simulink model "mpcController"  (R2022a)
settings: Solver=ode5  StartTime=0.0  StopTime=inf  RelTol=1e-3
values from neighbouring files (symbols this model uses):
  A_full = zeros(nX * (nH + 1), nX)    [controllerInit.m]
  B_full = zeros(nX * nH, nU * nH)    [controllerInit.m]
  lb_u_full = ub_u_full    [controllerInit.m]
  lb_x_full = ub_x_full    [controllerInit.m]
  opts = readyFamiliarisation(opts)    [main.m]
  R_full = zeros(nU * nH)    [controllerInit.m]
  ub_u_full = zeros(nU * nH, 1)    [controllerInit.m]
  ub_x_full = zeros(nX * (nH + 1), 1)    [controllerInit.m]
undefined symbols (not defined in the file or in its folder): C_full, QstructInitial, R_full_zeros, Serial_Port, simulinkStructInitial, Standard_Devices, UDP_Protocol
libraries: sldrtlib x5, simulink_extras x1, sharedtransform x1
settings Model: PacingRate=0.350000  Creator=simonas  LastModifiedBy=Simonas
settings HardwareCC: ProdBitPerLong=64  ProdHWDeviceType=Intel->x86-64 (Linux 64)
settings RTWCC: Description=Simulink Desktop Real-Time  SystemTargetFile=sldrt.tlc  TemplateMakefile=sldrt.tmf  RTWCompilerOptimization=on
settings CodeAppCC: MaxIdLength=95
settings SimulinkDesktopRealTimeCC: TargetLibSuffix=_sldrt.a  TargetPreCompLibLocation=C:\Program Files\MATLAB\R2022a\toolbox\sldrt\lib\win64

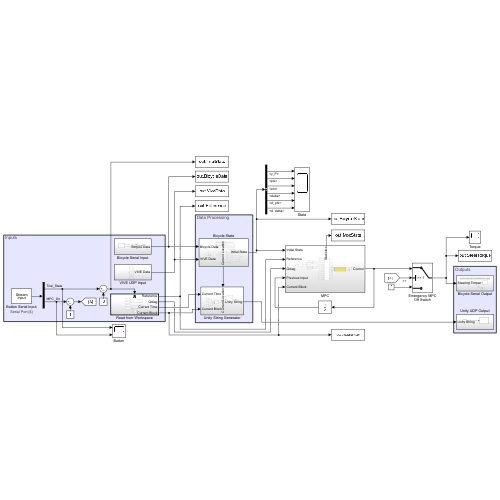
[thumbnail: Simulink's stored preview of the top-level diagram]
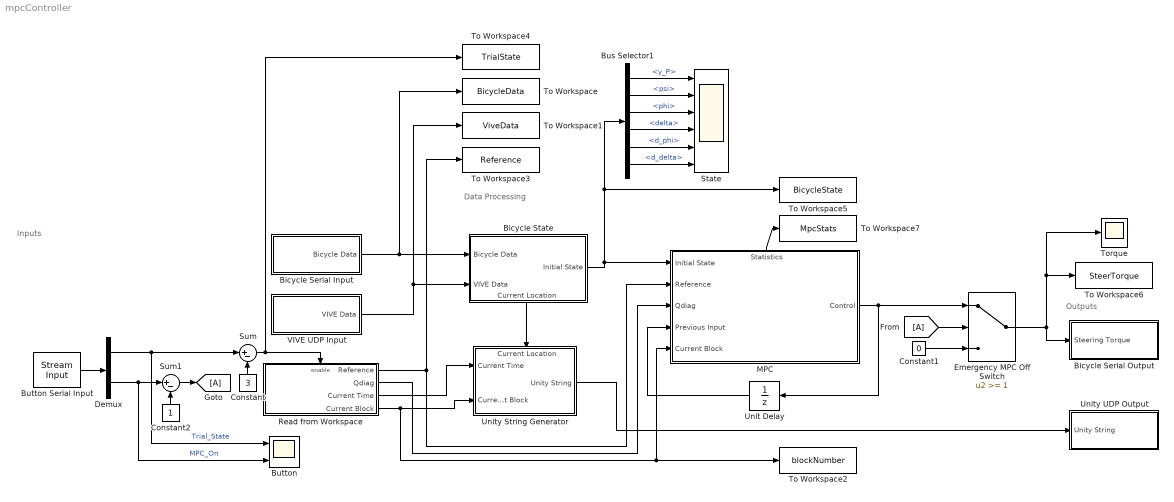
== system mpcController ==
  note: Inputs
  note: Data Processing
  note: Outputs
  Bicycle Serial Input : Subsystem
  Bicycle Serial Output : Subsystem
  Bicycle State : Subsystem
      settings: PortSchema="{\"entries\":[{\"content\":{\"sides\":[{\"content\":{\"connectorIds\":[\"In1\",\"In2\"]},\"type\":\"ConnectorPlacement.EquallySpacedRectSide\",\"uuid\":\"c5d89f74-e35e-400b-a49a-6a7c3bbb3cee\"},{\"content\":{\"connectorIds\":[\"Out1\"],\"side\":\"RIGHT\"},\"type\":\"ConnectorPlacement.EquallySpacedRectSide\",\"uuid\":\"d3946c1d-493c-4283-9feb-9c130facb0a9\"},{\"content\":{\"connectorIds\":[],\"side\":\"TOP\"},\"type\":\"ConnectorPlacement.EquallySpacedRectSide\",\"uuid\":\"f7eeef6e-15d0-4138-b893-66df70237323\"},{\"content\":{\"connectorIds\":[\"Out2\"],\"side\":\"BOTTOM\"},\"type\":\"ConnectorPlacement.EquallySpacedRectSide\",\"uuid\":\"d8cc5cfa-3fb7-476d-9b2c-860b356f327e\"}]},\"type\":\"ConnectorPlacement.EquallySpacedConnector\",\"uuid\":\"85360968-76db-44cc-98f9-7355ff2a9269\"}],\"packageUris\":[\"http://schema.mathworks.com/mf0/Connector/R2020b\"],\"version\":\"1.0\"}"
  Bus Selector1 : BusSelector  OutputSignals=y_P,psi,phi,delta,d_phi,d_delta
  Button : Scope  NumInputPorts=2
  Button Serial Input : sldrtlib/Stream Input  SampleTime=0.025  MaxMissedTicks=1000000  ShowMissedTicks=off  YieldWhenWaiting=off  DrvName=Standard_Devices/Serial_Port  DrvAddress=4  DrvOptions=[115200 8 0 0 0 0 0 0]  DataTypes='2*int32'  FormatString='%d,%d'  Terminator={'\n', '\r'}  ShowReady=off  ShowError=off
      settings: AttributesFormatString=Serial Port [4]  SourceProductBaseCode=WT
  Constant : Constant  Value=3
  Constant1 : Constant  Value=0  SampleTime=opts.Ts_mpc
  Constant2 : Constant
  Demux : Demux  Outputs=2
  Emergency MPC Off Switch : Switch  Threshold=1  SaturateOnIntegerOverflow=off  InputSameDT=off
  From : From
  Goto : Goto
  MPC : Subsystem
      settings: PortSchema="{\"entries\":[{\"content\":{\"sides\":[{\"content\":{\"connectorIds\":[\"In1\",\"In2\",\"In3\",\"In4\",\"In5\"]},\"type\":\"ConnectorPlacement.EquallySpacedRectSide\",\"uuid\":\"837940b0-492f-49e7-ad78-2f53a96cfdb0\"},{\"content\":{\"connectorIds\":[\"Out1\"],\"side\":\"RIGHT\"},\"type\":\"ConnectorPlacement.EquallySpacedRectSide\",\"uuid\":\"0b454771-57c7-4798-97e4-6e41a25b36dc\"},{\"content\":{\"connectorIds\":[\"Out2\"],\"side\":\"TOP\"},\"type\":\"ConnectorPlacement.EquallySpacedRectSide\",\"uuid\":\"d0d77e63-f0c6-441e-9a4a-b6dfb0057ad2\"},{\"content\":{\"connectorIds\":[],\"side\":\"BOTTOM\"},\"type\":\"ConnectorPlacement.EquallySpacedRectSide\",\"uuid\":\"b6921f02-8dc3-4ff1-8cb0-61ac83bc5ab1\"}]},\"type\":\"ConnectorPlacement.EquallySpacedConnector\",\"uuid\":\"6905a0a5-9fd3-4ab9-9143-61679843e617\"}],\"packageUris\":[\"http://schema.mathworks.com/mf0/Connector/R2020b\"],\"version\":\"1.0\"}"
  Read from Workspace : Subsystem  TreatAsAtomicUnit=on
  State : Scope  NumInputPorts=6
  Sum : Sum  Inputs=|+-
  Sum1 : Sum  Inputs=|+-
  To Workspace : ToWorkspace  VariableName=BicycleData  SaveFormat=Timeseries  SampleTime=-1
  To Workspace1 : ToWorkspace  VariableName=ViveData  SaveFormat=Timeseries  SampleTime=-1
  To Workspace2 : ToWorkspace  VariableName=blockNumber  SaveFormat=Timeseries  SampleTime=-1
  To Workspace3 : ToWorkspace  VariableName=Reference  SaveFormat=Timeseries  SampleTime=-1
  To Workspace4 : ToWorkspace  VariableName=TrialState  SaveFormat=Timeseries  SampleTime=-1
  To Workspace5 : ToWorkspace  VariableName=BicycleState  SaveFormat=Timeseries  SampleTime=-1
  To Workspace6 : ToWorkspace  VariableName=SteerTorque  SaveFormat=Timeseries  SampleTime=-1
  To Workspace7 : ToWorkspace  VariableName=MpcStats  SaveFormat=Timeseries  SampleTime=-1
  Torque : Scope
  Unit Delay : UnitDelay  SampleTime=opts.Ts_mpc  HasFrameUpgradeWarning=on
  Unity String Generator : Subsystem
      settings: PortSchema="{\"entries\":[{\"content\":{\"sides\":[{\"content\":{\"connectorIds\":[\"In1\",\"In2\"]},\"type\":\"ConnectorPlacement.EquallySpacedRectSide\",\"uuid\":\"995dcb62-78f8-423c-99d5-aa9c538d86ef\"},{\"content\":{\"connectorIds\":[\"Out1\"],\"side\":\"RIGHT\"},\"type\":\"ConnectorPlacement.EquallySpacedRectSide\",\"uuid\":\"d6e446ff-77b4-4bca-8c68-e505a29969fe\"},{\"content\":{\"connectorIds\":[\"In3\"],\"side\":\"TOP\"},\"type\":\"ConnectorPlacement.EquallySpacedRectSide\",\"uuid\":\"a2ee3f9a-5385-4b4c-abf0-7e00a59d14cf\"}]},\"type\":\"ConnectorPlacement.EquallySpacedConnector\",\"uuid\":\"6b026230-ac01-4f6d-82d7-753dc9fb2975\"}],\"packageUris\":[\"http://schema.mathworks.com/mf0/Connector/R2020b\"],\"version\":\"1.0\"}"
  Unity UDP Output : Subsystem
  VIVE UDP Input : Subsystem
  wires:
  Bicycle Serial Input/1(Bicycle Data) -> Bicycle State/1(Bicycle Data), To Workspace/1
  VIVE UDP Input/1(VIVE Data) -> Bicycle State/2(VIVE Data), To Workspace1/1
  Bicycle State/2(Current Location) -> Unity String Generator/3(Current Location)
  Bicycle State/1(Initial State) -> Bus Selector1/1, To Workspace5/1, MPC/1(Initial State)
  Demux/1 -> Sum/1, Button/1  "Trial_State"
  Button Serial Input/1 -> Demux/1
  Sum/1 -> To Workspace4/1, Read from Workspace/Enable
  Constant/1 -> Sum/2
  From/1 -> Emergency MPC Off Switch/2
  Constant1/1 -> Emergency MPC Off Switch/3
  Emergency MPC Off Switch/1 -> Bicycle Serial Output/1(Steering Torque), Torque/1, To Workspace6/1
  Sum1/1 -> Goto/1
  Constant2/1 -> Sum1/2
  Demux/2 -> Button/2, Sum1/1  "MPC_On"
  Read from Workspace/3(Current Time) -> Unity String Generator/1(Current Time)
  Read from Workspace/1(Reference) -> To Workspace3/1, MPC/2(Reference)
  Read from Workspace/2(Qdiag) -> MPC/3(Qdiag)
  MPC/2(Statistics) -> To Workspace7/1
  Unit Delay/1 -> MPC/4(Previous Input)
  Unity String Generator/1(Unity String) -> Unity UDP Output/1(Unity String)
  Bus Selector1/1 -> State/1  "<y_P>"
  Bus Selector1/3 -> State/3  "<phi>"
  Bus Selector1/4 -> State/4  "<delta>"
  Bus Selector1/2 -> State/2  "<psi>"
  Bus Selector1/5 -> State/5  "<d_phi>"
  Bus Selector1/6 -> State/6  "<d_delta>"
  MPC/1(Control) -> Emergency MPC Off Switch/1, Unit Delay/1
  Read from Workspace/4(Current Block) -> Unity String Generator/2(Current Block), MPC/5(Current Block), To Workspace2/1

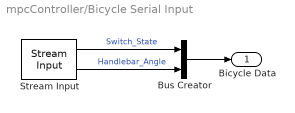
== system mpcController/Bicycle Serial Input ==
  Bus Creator : BusCreator  Inputs=2
  Stream Input : sldrtlib/Stream Input  SampleTime=opts.Ts_ser  MaxMissedTicks=1000000  ShowMissedTicks=off  YieldWhenWaiting=on  DrvName=Standard_Devices/Serial_Port  DrvAddress=3  DrvOptions=[115200 8 0 0 0 0 0 0]  DataTypes={'uint8','double'}  FormatString='%d,%f'  Terminator={'\n'}  ShowReady=off  ShowError=off
      settings: AttributesFormatString=Serial Port [3]  SourceProductBaseCode=WT
  Bicycle Data : Outport
  wires:
  Stream Input/1 -> Bus Creator/1  "Switch_State"
  Stream Input/2 -> Bus Creator/2  "Handlebar_Angle"
  Bus Creator/1 -> Bicycle Data/1

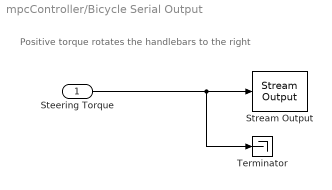
== system mpcController/Bicycle Serial Output ==
  note: Positive torque rotates the handlebars to the right
  Steering Torque : Inport
  Stream Output : sldrtlib/Stream Output  SampleTime=opts.Ts_mpc  MaxMissedTicks=1000000  ShowMissedTicks=off  YieldWhenWaiting=on  DrvName=Standard_Devices/Serial_Port  DrvAddress=3  DrvOptions=[115200 8 0 0 0 0 0 0]  PortSizes=1  FormatString='%.3f\n'  ShowReady=off  ShowError=off  InitialValue=[]  FinalValue=[]
      settings: AttributesFormatString=Serial Port [3]  SourceProductBaseCode=WT
  Terminator : Terminator
  wires:
  Steering Torque/1 -> Stream Output/1, Terminator/1

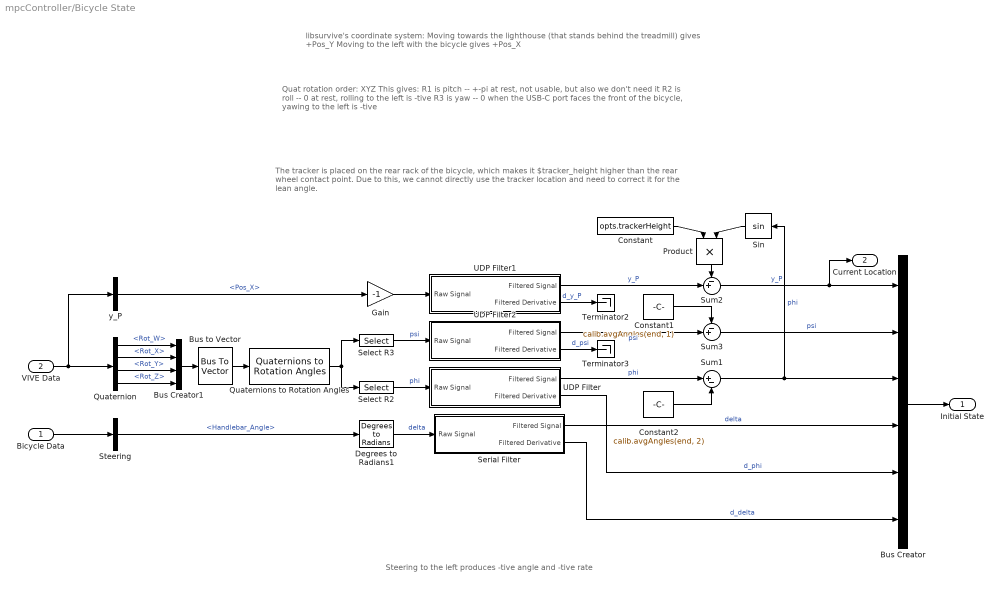
== system mpcController/Bicycle State ==
  note: The tracker is placed on the rear rack of the bicycle, which makes it $tracker_height higher than the rear wheel contact point. Due to this, we cannot directly use the tracker location and need to correct it for the lean angle.
  note: Steering to the left produces -tive angle and -tive rate
  note: libsurvive's coordinate system:
      | Moving towards the lighthouse (that stands behind the treadmill) gives +Pos_Y
      | Moving to the left with the bicycle gives +Pos_X
  note: Quat rotation order: XYZ
      | This gives:
      | R1 is pitch -- +-pi at rest, not usable, but also we don't need it
      | R2 is roll -- 0 at rest, rolling to the left is -tive
      | R3 is yaw -- 0 when the USB-C port faces the front of the bicycle, yawing to the left is -tive
  Bicycle Data : Inport
  VIVE Data : Inport  Port=2
  Bus Creator : BusCreator  Inputs=6
  Bus Creator1 : BusCreator  Inputs=4
  Bus to Vector : BusToVector
  Constant : Constant  Value=opts.trackerHeight
  Constant1 : Constant  Value=calib.avgAngles(end, 1)  SampleTime=opts.Ts_udp
  Constant2 : Constant  Value=calib.avgAngles(end, 2)  SampleTime=opts.Ts_udp
  Degrees to Radians1 : simulink_extras/Transformations/Degrees to Radians
  Gain : Gain  Gain=-1
  Product : Product
  Quaternion : BusSelector  OutputSignals=Rot_W,Rot_X,Rot_Y,Rot_Z
  Quaternions to Rotation Angles : sharedtransform/Quaternions to Rotation Angles  rotationOrder=XYZ  aMode=aMode
      settings: SourceProductBaseCode=AE,PW,DR,MT,VE
  Select R2 : Selector  InputPortWidth=3  IndexOptions=Index vector (dialog)  Indices=2  OutputSizes=1
  Select R3 : Selector  InputPortWidth=3  IndexOptions=Index vector (dialog)  Indices=3  OutputSizes=1
  Serial Filter : Subsystem
  Sin : Trigonometry
  Steering : BusSelector  OutputSignals=Handlebar_Angle
  Sum1 : Sum  Inputs=|+-
  Sum2 : Sum  Inputs=-+|
  Sum3 : Sum  Inputs=-+|
  Terminator2 : Terminator
  Terminator3 : Terminator
  UDP Filter : Subsystem
  UDP Filter1 : Subsystem
  UDP Filter2 : Subsystem
  y_P : BusSelector  OutputSignals=Pos_X
  Initial State : Outport
  Current Location : Outport  Port=2
  wires:
  VIVE Data/1 -> y_P/1, Quaternion/1
  Quaternion/2 -> Bus Creator1/2  "<Rot_X>"
  Quaternion/3 -> Bus Creator1/3  "<Rot_Y>"
  Quaternion/4 -> Bus Creator1/4  "<Rot_Z>"
  Select R2/1 -> UDP Filter/1(Raw Signal)  "phi"
  y_P/1 -> Gain/1  "<Pos_X>"
  Bicycle Data/1 -> Steering/1
  Steering/1 -> Degrees to Radians1/1  "<Handlebar_Angle>"
  Bus Creator/1 -> Initial State/1
  Quaternion/1 -> Bus Creator1/1  "<Rot_W>"
  Bus Creator1/1 -> Bus to Vector/1
  Bus to Vector/1 -> Quaternions to Rotation Angles/1
  Quaternions to Rotation Angles/1 -> Select R3/1, Select R2/1
  Degrees to Radians1/1 -> Serial Filter/1(Raw Signal)  "delta"
  Gain/1 -> UDP Filter1/1(Raw Signal)
  Constant/1 -> Product/1
  Sin/1 -> Product/2
  UDP Filter/2(Filtered Derivative) -> Bus Creator/5  "d_phi"
  Serial Filter/1(Filtered Signal) -> Bus Creator/4  "delta"
  Serial Filter/2(Filtered Derivative) -> Bus Creator/6  "d_delta"
  UDP Filter1/2(Filtered Derivative) -> Terminator2/1  "d_y_P"
  Select R3/1 -> UDP Filter2/1(Raw Signal)  "psi"
  UDP Filter2/1(Filtered Signal) -> Sum3/2  "psi"
  UDP Filter2/2(Filtered Derivative) -> Terminator3/1  "d_psi"
  UDP Filter1/1(Filtered Signal) -> Sum2/2  "y_P"
  Sum2/1 -> Current Location/1, Bus Creator/1  "y_P"
  Product/1 -> Sum2/1
  Sum1/1 -> Sin/1, Bus Creator/3  "phi"
  Sum3/1 -> Bus Creator/2  "psi"
  Constant1/1 -> Sum3/1
  UDP Filter/1(Filtered Signal) -> Sum1/1  "phi"
  Constant2/1 -> Sum1/2

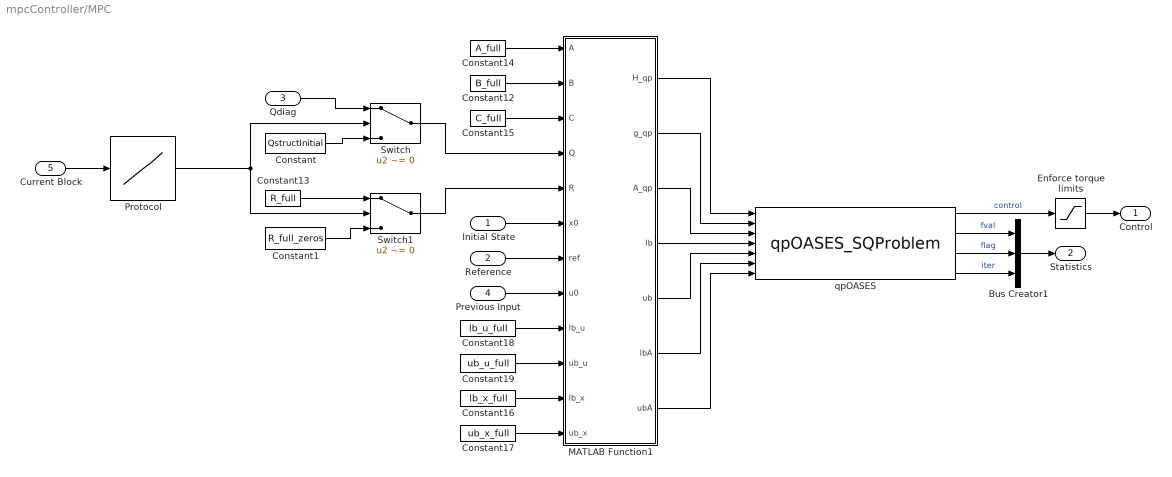
== system mpcController/MPC ==
  Initial State : Inport
  Reference : Inport  Port=2
  Qdiag : Inport  Port=3
  Previous Input : Inport  Port=4
  Current Block : Inport  Port=5
  Bus Creator1 : BusCreator  Inputs=3
  Constant : Constant  Value=QstructInitial
  Constant1 : Constant  Value=R_full_zeros  SampleTime=opts.Ts_mpc
  Constant12 : Constant  Value=B_full  SampleTime=opts.Ts_mpc
  Constant13 : Constant  Value=R_full  SampleTime=opts.Ts_mpc
  Constant14 : Constant  Value=A_full  SampleTime=opts.Ts_mpc
  Constant15 : Constant  Value=C_full  SampleTime=opts.Ts_mpc
  Constant16 : Constant  Value=lb_x_full  SampleTime=opts.Ts_mpc
  Constant17 : Constant  Value=ub_x_full  SampleTime=opts.Ts_mpc
  Constant18 : Constant  Value=lb_u_full  SampleTime=opts.Ts_mpc
  Constant19 : Constant  Value=ub_u_full  SampleTime=opts.Ts_mpc
  Enforce torque limits : Saturate  UpperLimit=opts.steerTorqueLim  LowerLimit=-opts.steerTorqueLim
  MATLAB Function1 : MATLAB Function  TreatAsAtomicUnit=on  SystemSampleTime=opts.Ts_mpc  VariantControl=Choice
  Protocol : Lookup_n-D  NumberOfTableDimensions=1  BreakpointsForDimension1=opts.lookupBreakpoints  Table=opts.lookupValues  InternalRulePriority=Speed  RndMeth=Simplest
  Switch : Switch  Criteria=u2 ~= 0  SaturateOnIntegerOverflow=off  InputSameDT=off
  Switch1 : Switch  Criteria=u2 ~= 0  SaturateOnIntegerOverflow=off  InputSameDT=off
  qpOASES : S-Function  FunctionName=qpOASES_SQProblem  SFunctionDeploymentMode=off  EnableBusSupport=off
  Control : Outport
  Statistics : Outport  Port=2
  wires:
  Enforce torque limits/1 -> Control/1
  Constant12/1 -> MATLAB Function1/2(B)
  Constant18/1 -> MATLAB Function1/9(lb_u)
  MATLAB Function1/1(H_qp) -> qpOASES/1
  Constant16/1 -> MATLAB Function1/11(lb_x)
  Constant19/1 -> MATLAB Function1/10(ub_u)
  Constant17/1 -> MATLAB Function1/12(ub_x)
  Bus Creator1/1 -> Statistics/1
  qpOASES/4 -> Bus Creator1/3  "iter"
  qpOASES/2 -> Bus Creator1/1  "fval"
  MATLAB Function1/3(A_qp) -> qpOASES/3
  Reference/1 -> MATLAB Function1/7(ref)
  qpOASES/3 -> Bus Creator1/2  "flag"
  MATLAB Function1/4(lb) -> qpOASES/4
  MATLAB Function1/2(g_qp) -> qpOASES/2
  Constant14/1 -> MATLAB Function1/1(A)
  MATLAB Function1/5(ub) -> qpOASES/5
  MATLAB Function1/7(ubA) -> qpOASES/7
  Constant15/1 -> MATLAB Function1/3(C)
  MATLAB Function1/6(lbA) -> qpOASES/6
  Previous Input/1 -> MATLAB Function1/8(u0)
  Initial State/1 -> MATLAB Function1/6(x0)
  qpOASES/1 -> Enforce torque limits/1  "control"
  Current Block/1 -> Protocol/1
  Switch/1 -> MATLAB Function1/4(Q)
  Qdiag/1 -> Switch/1
  Switch1/1 -> MATLAB Function1/5(R)
  Constant13/1 -> Switch1/1
  Protocol/1 -> Switch1/2, Switch/2
  Constant/1 -> Switch/3
  Constant1/1 -> Switch1/3

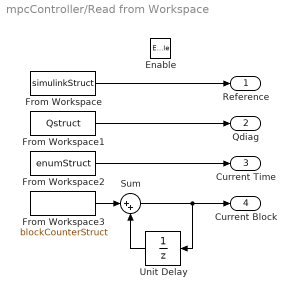
== system mpcController/Read from Workspace ==
  Enable : EnablePort  StatesWhenEnabling=reset
  From Workspace : FromWorkspace  VariableName=simulinkStruct  SampleTime=opts.Ts_mpc  Interpolate=off  OutputAfterFinalValue=Cyclic repetition
  From Workspace1 : FromWorkspace  VariableName=Qstruct  SampleTime=opts.Ts_mpc  Interpolate=off  OutputAfterFinalValue=Cyclic repetition
  From Workspace2 : FromWorkspace  VariableName=enumStruct  SampleTime=opts.Ts_mpc  Interpolate=off  OutputAfterFinalValue=Cyclic repetition
  From Workspace3 : FromWorkspace  VariableName=blockCounterStruct  SampleTime=opts.Ts_mpc  Interpolate=off  OutputAfterFinalValue=Cyclic repetition
  Sum : Sum  Inputs=|++
  Unit Delay : UnitDelay  InitialCondition=1  SampleTime=opts.Ts_mpc  HasFrameUpgradeWarning=on
  Reference : Outport  InitialOutput=simulinkStructInitial
  Qdiag : Outport  Port=2  OutputWhenDisabled=reset  InitialOutput=QstructInitial
  Current Time : Outport  Port=3  OutputWhenDisabled=reset  InitialOutput=0
  Current Block : Outport  Port=4  OutputWhenDisabled=reset  InitialOutput=1
  wires:
  From Workspace/1 -> Reference/1
  From Workspace1/1 -> Qdiag/1
  From Workspace2/1 -> Current Time/1
  From Workspace3/1 -> Sum/1
  Sum/1 -> Unit Delay/1, Current Block/1
  Unit Delay/1 -> Sum/2

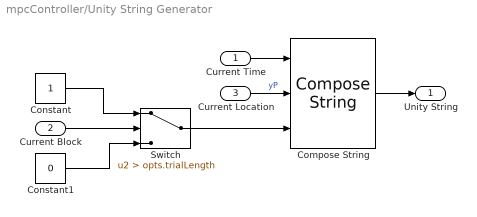
== system mpcController/Unity String Generator ==
  Current Time : Inport
  Current Block : Inport  Port=2
  Current Location : Inport  Port=3
  Compose String : ComposeString  Format="\"%.0f,%.3f,%.0f\\n\""
  Constant : Constant
  Constant1 : Constant  Value=0
  Switch : Switch  Criteria=u2 > Threshold  Threshold=opts.trialLength  SaturateOnIntegerOverflow=off  InputSameDT=off
  Unity String : Outport  OutDataTypeStr=string
  wires:
  Current Time/1 -> Compose String/1
  Current Location/1 -> Compose String/2  "yP"
  Compose String/1 -> Unity String/1
  Current Block/1 -> Switch/2
  Constant/1 -> Switch/1
  Constant1/1 -> Switch/3
  Switch/1 -> Compose String/3

== system mpcController/Unity UDP Output ==
  Unity String : Inport
  Stream Output : sldrtlib/Stream Output  SampleTime=opts.Ts_udp  MaxMissedTicks=1000000  ShowMissedTicks=off  YieldWhenWaiting=on  DrvName=Standard_Devices/UDP_Protocol  DrvAddress=8005  DrvOptions=[0 8006 49 50 55 46 48 46 48 46 49 0 0 0 0 0 0 0 0 0 0 0 0 0 0 0 0 0 0 0 0 0 0 0 0 0 0 0 0 0 0 0 0 0 0 0 0 0 0 0 0 0 0 0 0 0 0 0 0 0 0 0 0 0 0 0 0 0 0 0 0 0 0 0 0 0 0 0 0 0 0 0 0 0 0 0 0 0 0 0 0 0 0 0 0 0 0 0 0 0 0 0 0 0 0 0 0 0 0 0 0 0 0 0 0 0 0 0 0 0 0 0 0 0 0 0 0 0 0 0 0 0 0 0 0 0 0 0 0 0 0 0 0 0 0 0 0 0 0 0 0 0 0 0 0 0 0 0 0 0 0 0 0 0 0 0 0 0 0 0 0 0 0 0 0 0 0 0 0 0 0 0 0 0 0 0 0 0 0 0 0 0 0 0 0 0 0 0 0 0 0 0 0 0 0 0 0 0 0 0 0 0 0 0 0 0 0 0 0 0 0 0 0 0 0 0 0 0 0 0 0 0 0 0 0 0 0 0 0 0 0 0 0 0 0 0 0 0 0 0 0 0 0 0 0 0]  PortSizes=1  FormatString='%s'  ShowReady=off  ShowError=off  InitialValue=[]  FinalValue=[]
      settings: AttributesFormatString=UDP Protocol [8005]  SourceProductBaseCode=WT
  wires:
  Unity String/1 -> Stream Output/1

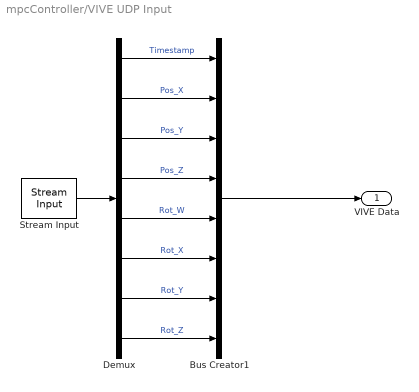
== system mpcController/VIVE UDP Input ==
  Bus Creator1 : BusCreator  Inputs=8
  Demux : Demux  Outputs=8
  Stream Input : sldrtlib/Stream Input  SampleTime=opts.Ts_udp  MaxMissedTicks=1000000  ShowMissedTicks=off  YieldWhenWaiting=on  DrvName=Standard_Devices/UDP_Protocol  DrvAddress=4950  DrvOptions=[0 16385 0 0 0 0 0 0 0 0 0 0 0 0 0 0 0 0 0 0 0 0 0 0 0 0 0 0 0 0 0 0 0 0 0 0 0 0 0 0 0 0 0 0 0 0 0 0 0 0 0 0 0 0 0 0 0 0 0 0 0 0 0 0 0 0 0 0 0 0 0 0 0 0 0 0 0 0 0 0 0 0 0 0 0 0 0 0 0 0 0 0 0 0 0 0 0 0 0 0 0 0 0 0 0 0 0 0 0 0 0 0 0 0 0 0 0 0 0 0 0 0 0 0 0 0 0 0 0 0 0 0 0 0 0 0 0 0 0 0 0 0 0 0 0 0 0 0 0 0 0 0 0 0 0 0 0 0 0 0 0 0 0 0 0 0 0 0 0 0 0 0 0 0 0 0 0 0 0 0 0 0 0 0 0 0 0 0 0 0 0 0 0 0 0 0 0 0 0 0 0 0 0 0 0 0 0 0 0 0 0 0 0 0 0 0 0 0 0 0 0 0 0 0 0 0 0 0 0 0 0 0 0 0 0 0 0 0 0 0 0 0 0 0 0 0 0 0 0 0 0 0 0 0 0 0]  DataTypes={'8*double'}  FormatString='%f,%f,%f,%f,%f,%f,%f,%f'  Terminator='\n'  ShowReady=off  ShowError=off
      settings: AttributesFormatString=UDP Protocol [4950]  SourceProductBaseCode=WT
  VIVE Data : Outport
  wires:
  Demux/4 -> Bus Creator1/4  "Pos_Z"
  Demux/5 -> Bus Creator1/5  "Rot_W"
  Demux/7 -> Bus Creator1/7  "Rot_Y"
  Demux/6 -> Bus Creator1/6  "Rot_X"
  Demux/1 -> Bus Creator1/1  "Timestamp"
  Demux/2 -> Bus Creator1/2  "Pos_X"
  Demux/8 -> Bus Creator1/8  "Rot_Z"
  Demux/3 -> Bus Creator1/3  "Pos_Y"
  Bus Creator1/1 -> VIVE Data/1
  Stream Input/1 -> Demux/1

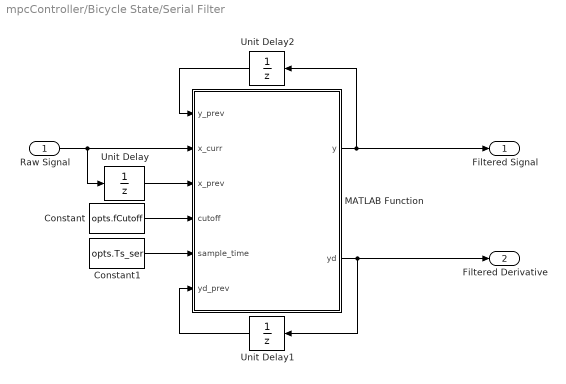
== system mpcController/Bicycle State/Serial Filter ==
  Raw Signal : Inport
  Constant : Constant  Value=opts.fCutoff  SampleTime=opts.Ts_ser
  Constant1 : Constant  Value=opts.Ts_ser  SampleTime=opts.Ts_ser
  MATLAB Function : MATLAB Function  TreatAsAtomicUnit=on
  Unit Delay : UnitDelay  SampleTime=opts.Ts_ser  HasFrameUpgradeWarning=on
  Unit Delay1 : UnitDelay  SampleTime=opts.Ts_ser  HasFrameUpgradeWarning=on
  Unit Delay2 : UnitDelay  SampleTime=opts.Ts_ser  HasFrameUpgradeWarning=on
  Filtered Signal : Outport
  Filtered Derivative : Outport  Port=2
  wires:
  MATLAB Function/1(y) -> Unit Delay2/1, Filtered Signal/1
  MATLAB Function/2(yd) -> Unit Delay1/1, Filtered Derivative/1
  Raw Signal/1 -> Unit Delay/1, MATLAB Function/2(x_curr)
  Unit Delay/1 -> MATLAB Function/3(x_prev)
  Constant/1 -> MATLAB Function/4(cutoff)
  Constant1/1 -> MATLAB Function/5(sample_time)
  Unit Delay2/1 -> MATLAB Function/1(y_prev)
  Unit Delay1/1 -> MATLAB Function/6(yd_prev)

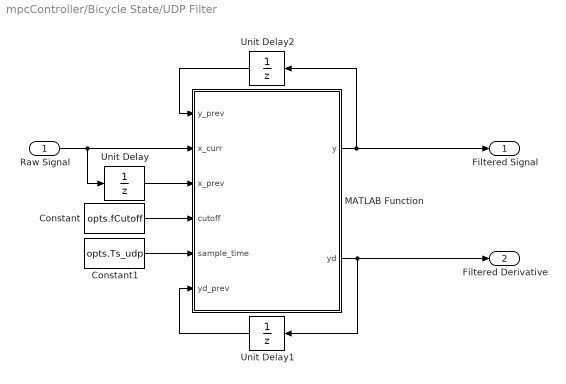
== system mpcController/Bicycle State/UDP Filter ==
  Raw Signal : Inport
  Constant : Constant  Value=opts.fCutoff  SampleTime=opts.Ts_udp
  Constant1 : Constant  Value=opts.Ts_udp  SampleTime=opts.Ts_udp
  MATLAB Function : MATLAB Function  TreatAsAtomicUnit=on
  Unit Delay : UnitDelay  SampleTime=opts.Ts_udp  HasFrameUpgradeWarning=on
  Unit Delay1 : UnitDelay  SampleTime=opts.Ts_udp  HasFrameUpgradeWarning=on
  Unit Delay2 : UnitDelay  SampleTime=opts.Ts_udp  HasFrameUpgradeWarning=on
  Filtered Signal : Outport
  Filtered Derivative : Outport  Port=2
  wires:
  MATLAB Function/1(y) -> Unit Delay2/1, Filtered Signal/1
  MATLAB Function/2(yd) -> Unit Delay1/1, Filtered Derivative/1
  Raw Signal/1 -> Unit Delay/1, MATLAB Function/2(x_curr)
  Unit Delay/1 -> MATLAB Function/3(x_prev)
  Constant/1 -> MATLAB Function/4(cutoff)
  Constant1/1 -> MATLAB Function/5(sample_time)
  Unit Delay2/1 -> MATLAB Function/1(y_prev)
  Unit Delay1/1 -> MATLAB Function/6(yd_prev)

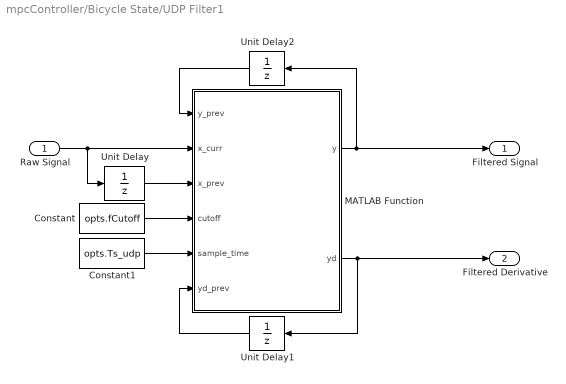
== system mpcController/Bicycle State/UDP Filter1 ==
  Raw Signal : Inport
  Constant : Constant  Value=opts.fCutoff  SampleTime=opts.Ts_udp
  Constant1 : Constant  Value=opts.Ts_udp  SampleTime=opts.Ts_udp
  MATLAB Function : MATLAB Function  TreatAsAtomicUnit=on
  Unit Delay : UnitDelay  SampleTime=opts.Ts_udp  HasFrameUpgradeWarning=on
  Unit Delay1 : UnitDelay  SampleTime=opts.Ts_udp  HasFrameUpgradeWarning=on
  Unit Delay2 : UnitDelay  SampleTime=opts.Ts_udp  HasFrameUpgradeWarning=on
  Filtered Signal : Outport
  Filtered Derivative : Outport  Port=2
  wires:
  MATLAB Function/1(y) -> Unit Delay2/1, Filtered Signal/1
  MATLAB Function/2(yd) -> Unit Delay1/1, Filtered Derivative/1
  Raw Signal/1 -> Unit Delay/1, MATLAB Function/2(x_curr)
  Unit Delay/1 -> MATLAB Function/3(x_prev)
  Constant/1 -> MATLAB Function/4(cutoff)
  Constant1/1 -> MATLAB Function/5(sample_time)
  Unit Delay2/1 -> MATLAB Function/1(y_prev)
  Unit Delay1/1 -> MATLAB Function/6(yd_prev)

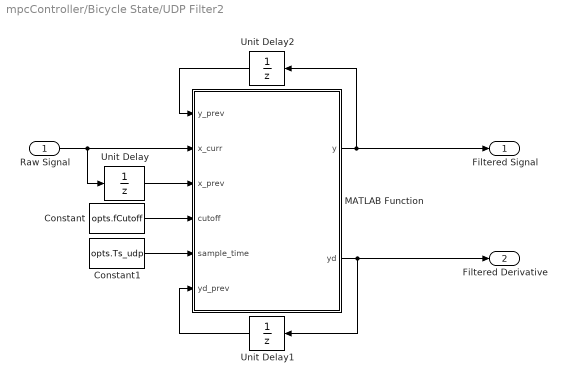
== system mpcController/Bicycle State/UDP Filter2 ==
  Raw Signal : Inport
  Constant : Constant  Value=opts.fCutoff  SampleTime=opts.Ts_udp
  Constant1 : Constant  Value=opts.Ts_udp  SampleTime=opts.Ts_udp
  MATLAB Function : MATLAB Function  TreatAsAtomicUnit=on
  Unit Delay : UnitDelay  SampleTime=opts.Ts_udp  HasFrameUpgradeWarning=on
  Unit Delay1 : UnitDelay  SampleTime=opts.Ts_udp  HasFrameUpgradeWarning=on
  Unit Delay2 : UnitDelay  SampleTime=opts.Ts_udp  HasFrameUpgradeWarning=on
  Filtered Signal : Outport
  Filtered Derivative : Outport  Port=2
  wires:
  MATLAB Function/1(y) -> Unit Delay2/1, Filtered Signal/1
  MATLAB Function/2(yd) -> Unit Delay1/1, Filtered Derivative/1
  Raw Signal/1 -> Unit Delay/1, MATLAB Function/2(x_curr)
  Unit Delay/1 -> MATLAB Function/3(x_prev)
  Constant/1 -> MATLAB Function/4(cutoff)
  Constant1/1 -> MATLAB Function/5(sample_time)
  Unit Delay2/1 -> MATLAB Function/1(y_prev)
  Unit Delay1/1 -> MATLAB Function/6(yd_prev)

== matlab function mpcController/Bicycle State/UDP Filter/MATLAB Function ==
  data: y_prev input; y output; x_curr input; x_prev input; cutoff input; sample_time input; yd_prev input; yd output
function [y, yd] = realtime_filter(y_prev, x_curr, x_prev, ...
                                   cutoff, sample_time, yd_prev)
a = (2*pi * cutoff^2);
b = sqrt(2) * 2*pi * cutoff;
h = sample_time;
denom = 4 + 2*h*b + h^2*a;

A = (4 + 2*h*b - h^2*a) / denom;
B = 4*h / denom;
C = -4*h*a / denom;
D = (4 - 2*h*b - h^2*a) / denom;
E = 2*h^2*a / denom;
F = 4*h*a / denom;

y = A * y_prev + B * yd_prev + E * (x_curr + x_prev) / 2;
yd = C * y_prev + D * yd_prev + F * (x_curr + x_prev) / 2;

== matlab function mpcController/Bicycle State/Serial Filter/MATLAB Function ==
  data: y_prev input; y output; x_curr input; x_prev input; cutoff input; sample_time input; yd_prev input; yd output
function [y, yd] = realtime_filter(y_prev, x_curr, x_prev, ...
                                   cutoff, sample_time, yd_prev)
a = (2*pi * cutoff^2);
b = sqrt(2) * 2*pi * cutoff;
h = sample_time;
denom = 4 + 2*h*b + h^2*a;

A = (4 + 2*h*b - h^2*a) / denom;
B = 4*h / denom;
C = -4*h*a / denom;
D = (4 - 2*h*b - h^2*a) / denom;
E = 2*h^2*a / denom;
F = 4*h*a / denom;

y = A * y_prev + B * yd_prev + E * (x_curr + x_prev) / 2;
yd = C * y_prev + D * yd_prev + F * (x_curr + x_prev) / 2;

== matlab function mpcController/Bicycle State/UDP Filter1/MATLAB Function ==
  data: y_prev input; y output; x_curr input; x_prev input; cutoff input; sample_time input; yd_prev input; yd output
function [y, yd] = realtime_filter(y_prev, x_curr, x_prev, ...
                                   cutoff, sample_time, yd_prev)
a = (2*pi * cutoff^2);
b = sqrt(2) * 2*pi * cutoff;
h = sample_time;
denom = 4 + 2*h*b + h^2*a;

A = (4 + 2*h*b - h^2*a) / denom;
B = 4*h / denom;
C = -4*h*a / denom;
D = (4 - 2*h*b - h^2*a) / denom;
E = 2*h^2*a / denom;
F = 4*h*a / denom;

y = A * y_prev + B * yd_prev + E * (x_curr + x_prev) / 2;
yd = C * y_prev + D * yd_prev + F * (x_curr + x_prev) / 2;

== matlab function mpcController/Bicycle State/UDP Filter2/MATLAB Function ==
  data: y_prev input; y output; x_curr input; x_prev input; cutoff input; sample_time input; yd_prev input; yd output
function [y, yd] = realtime_filter(y_prev, x_curr, x_prev, ...
                                   cutoff, sample_time, yd_prev)
a = (2*pi * cutoff^2);
b = sqrt(2) * 2*pi * cutoff;
h = sample_time;
denom = 4 + 2*h*b + h^2*a;

A = (4 + 2*h*b - h^2*a) / denom;
B = 4*h / denom;
C = -4*h*a / denom;
D = (4 - 2*h*b - h^2*a) / denom;
E = 2*h^2*a / denom;
F = 4*h*a / denom;

y = A * y_prev + B * yd_prev + E * (x_curr + x_prev) / 2;
yd = C * y_prev + D * yd_prev + F * (x_curr + x_prev) / 2;

== matlab function mpcController/MPC/MATLAB Function1 ==
  data: H_qp output; g_qp output; A input; A_qp output; B input; C input; Q input; R input; x0 input; ref input; u0 input; lb_u input; ub_u input; lb_x input; ub_x input; lb output; ub output; lbA output; ubA output
function [H_qp, g_qp, A_qp, lb, ub, lbA, ubA] = fcn(A, B, C, Q, R, x0, ref, u0, lb_u, ub_u, lb_x, ub_x) %#codegen

temp = B' .* Q';
H = temp * B + R;

A_qp = B(:);
H_qp = H(:);
g_qp = [temp * A, ...
        -temp, ...
        temp * C] * [x0; ref; u0];

temp = - A * x0 - C * u0;

lb = lb_u;
ub = ub_u;
lbA = lb_x + temp;
ubA = ub_x + temp;
